simulink model "sim_quadrotor"  (R2015a)
settings: Solver=ode3  StartTime=0  StopTime=inf  FixedStep=quadEDT.sampletime  MaxStep=0.1  RelTol=1e-3
InitFcn:
  | % load parameters of the default quadrotor
  | disp('Quadrotor parameters loaded by InitFcn')
  | parameters_estimationcontrol %loads mdl_quadcopter, too!
  | 
  | % change to Simulation folder if in data folder
  | cd([matlabpath '/Simulation']);
undefined symbols (not defined in the file or in its folder): controlHelperParams, Discrete, estimParams, quad, quadEDT, Time
libraries: simulink x30, ctrlSharedLib x3, vrlib x1, commnoisgen2 x1, aerolibtransform2 x1
(part 1 of 2)
settings Model: CovSFcnEnable=off  Creator=corkep  LastModifiedBy=ra
settings DataIOCC: LimitDataPoints=off  SaveFormat=StructureWithTime  SignalLoggingSaveFormat=ModelDataLogs  SignalLogging=off  DSMLogging=off
settings OptimizationCC: ExpressionDepthLimit=2147483647  OptimizeModelRefInitCode=on  LifeSpan=1
settings DebuggingCC: UnderspecifiedInitializationDetection=Classic  MergeDetectMultiDrivingBlocksExec=none  SolverPrmCheckMsg=warning  FcnCallInpInsideContextMsg=UseLocalSettings  StateNameClashWarn=warning
settings HardwareCC: TargetBitPerLong=64  TargetBitPerPointer=64  TargetLongLongMode=on  TargetIntDivRoundTo=Zero  TargetEndianess=LittleEndian  TargetWordSize=64  TargetHWDeviceType=MATLAB Host  ProdEqTarget=off
settings RTWCC: SystemTargetFile=ert_shrlib.tlc  GenCodeOnly=on  MakeCommand="make_rtw OPTS=\"-DDEFAULT_BUFFER_SIZE=4600\""  GenerateMakefile=off  TemplateMakefile=ert_default_tmf  Description=Embedded Coder (host-based shared library target)  BuildConfiguration=Faster Runs  RTWCompilerOptimization=on
settings CodeAppCC: IgnoreCustomStorageClasses=off
settings STFCustomTargetCC: ParMdlRefBuildCompliant=on  CompOptLevelCompliant=on  IncludeMdlTerminateFcn=off  CombineOutputUpdateFcns=on  MultiInstanceERTCode=on  CodeInterfacePackaging=Reusable function  SupportVariableSizeSignals=off  ModelStepFunctionPrototypeControlCompliant=on  SystemTargetFile=ert_shrlib.tlc
settings ERTTargetCC: ParMdlRefBuildCompliant=on  CompOptLevelCompliant=on  IncludeMdlTerminateFcn=off  MultiInstanceERTCode=on  CodeInterfacePackaging=Reusable function  SupportVariableSizeSignals=off  ModelStepFunctionPrototypeControlCompliant=on  MultiInstanceErrorCode=Warning  ERTCustomFileTemplate=example_file_process.tlc

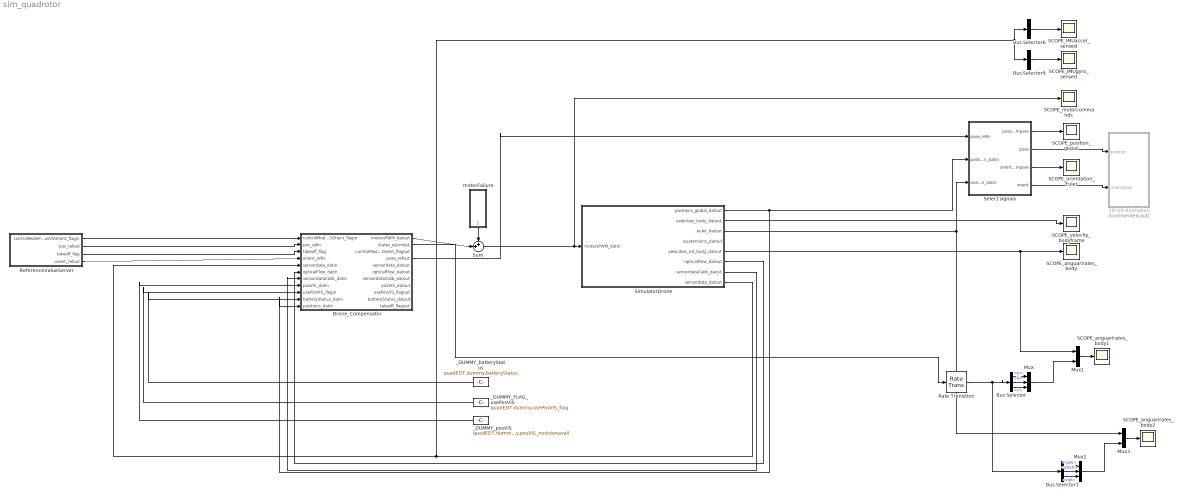
== system sim_quadrotor ==
  3D-VR-Animation : Subsystem  Commented=on
  Bus Selector : BusSelector  OutputSignals=p,q,r
  Bus Selector1 : BusSelector  OutputSignals=yaw,pitch,roll
  Bus Selector6 : BusSelector  OutputSignals=ddx,ddy,ddz  OutputAsBus=on
  Bus Selector9 : BusSelector  OutputSignals=p,q,r  OutputAsBus=on
  Drone_Compensator : Subsystem  TreatAsAtomicUnit=on
  Mux : Mux  Inputs=3
  Mux1 : Mux  Inputs=2
  Mux2 : Mux  Inputs=3
  Mux3 : Mux  Inputs=2
  Rate Transition : RateTransition
  ReferenceValueServer : Subsystem
  SCOPE_IMUaccel_sensed : Scope
      settings: TimeRange=14.995  YMin=-13  YMax=2  SaveName=ScopeData11
  SCOPE_IMUgyro_sensed : Scope
      settings: TimeRange=14.995  YMin=-0.002  YMax=0.00175  SaveName=ScopeData10
  SCOPE_anguarlrates_body : Scope
      settings: TimeRange=13.045  YMin=-1.5  YMax=0.5  SaveName=ScopeData7
  SCOPE_anguarlrates_body1 : Scope
      settings: TimeRange=13.045  YMin=-1.5  YMax=0.5  SaveName=ScopeData8
  SCOPE_anguarlrates_body2 : Scope
      settings: TimeRange=13.045  YMin=-1.5  YMax=0.5  SaveName=ScopeData13
  SCOPE_motorcommands : Scope
      settings: TimeRange=20.435  YMin=1200  YMax=1450  SaveName=ScopeData2
  SCOPE_orientation_Euler : Scope
      settings: TimeRange=29.325  YMin=-0.1  YMax=0.15  SaveName=ScopeData5
  SCOPE_position_global : Scope
      settings: TimeRange=24.935  YMin=-1.5  YMax=1  SaveName=ScopeData3
  SCOPE_velocity_bodyframe : Scope
      settings: TimeRange=13.045  YMin=-1.5  YMax=0.5  SaveName=ScopeData22
  Select signals : Subsystem
  SimulatorDrone : Subsystem
  Sum : Sum  Inputs=++|
  _DUMMY_FLAG_usePosVIS : Constant  Value=quadEDT.dummy.usePosVIS_flag
  _DUMMY_batteryStatus : Constant  Value=quadEDT.dummy.batteryStatus
  _DUMMY_posVIS : Constant  Value=quadEDT.dummy.posVIS_novisionavail
  motorFailure : Subsystem
  wires:
  Bus Selector6/1 -> SCOPE_IMUaccel_sensed/1
  Bus Selector9/1 -> SCOPE_IMUgyro_sensed/1
  ReferenceValueServer/2("pos_refout ") -> Drone_Compensator/2(pos_refin)
  motorFailure/1(motors_datout) -> Sum/1
  Drone_Compensator/1(motorsPWM_datout) -> Sum/2
  ReferenceValueServer/1(controlModePosVSOrient_flagin) -> Drone_Compensator/1(controlModePosVSOrient_flagin)
  ReferenceValueServer/4(orient_refout) -> Drone_Compensator/4(orient_refin)
  _DUMMY_posVIS/1 -> Drone_Compensator/8(posVIS_datin)
  _DUMMY_FLAG_usePosVIS/1 -> Drone_Compensator/9(usePosVIS_flagin)
  _DUMMY_batteryStatus/1 -> Drone_Compensator/10(batteryStatus_datin)
  ReferenceValueServer/3("takeoff_flag ") -> Drone_Compensator/3(takeoff_flag)
  Drone_Compensator/4(pose_refout) -> Select signals/1(pose_refin)
  Select signals/1(poseCompare) -> SCOPE_position_global/1
  Select signals/2(pose) -> 3D-VR-Animation/1(position)
  Select signals/3(orientCompare) -> SCOPE_orientation_Euler/1
  Select signals/4(orient) -> 3D-VR-Animation/2(orientation)
  SimulatorDrone/8(sensordata_datout) -> Bus Selector9/1, Bus Selector6/1, Drone_Compensator/5(sensordata_datin)
  SimulatorDrone/6(opticalFlow_datout) -> Drone_Compensator/6(opticalFlow_datin)
  SimulatorDrone/7(sensordataCalib_daout) -> Drone_Compensator/7(sensordataCalib_datin)
  SimulatorDrone/1(positions_global_datout) -> Select signals/2(position_datin), Drone_Compensator/11(positions_datin)
  SimulatorDrone/2(velocities_body_datout) -> SCOPE_velocity_bodyframe/1
  SimulatorDrone/3(euler_datout) -> Mux3/1, Select signals/3(orientation_datin)
  SimulatorDrone/5(velocities_rot_body_datout) -> Mux1/1, SCOPE_anguarlrates_body/1
  Drone_Compensator/2(states_estimout) -> Rate Transition/1
  Bus Selector/1 -> Mux/1  "<p>"
  Bus Selector/2 -> Mux/2  "<q>"
  Bus Selector/3 -> Mux/3  "<r>"
  Mux/1 -> Mux1/2
  Mux1/1 -> SCOPE_anguarlrates_body1/1
  Rate Transition/1 -> Bus Selector1/1, Bus Selector/1
  Bus Selector1/1 -> Mux2/1  "<yaw>"
  Bus Selector1/2 -> Mux2/2  "<pitch>"
  Bus Selector1/3 -> Mux2/3  "<roll>"
  Mux2/1 -> Mux3/2
  Mux3/1 -> SCOPE_anguarlrates_body2/1
  Sum/1 -> SCOPE_motorcommands/1, SimulatorDrone/1(motorsPWM_datin)

== system sim_quadrotor/3D-VR-Animation ==
  note: Student contribution by Erlend Solbakk Harbitz
  note: In animation:
      | X-axis: red
      | Y-axis: green
      | Z-axis: blue
  note: Animation
  note: Positions = [X; Y; Z] (Inertia frame with Z-axis downwards)
      | Theta      = [yaw (psi); pitch ( theta); roll (phi) ]
      |
      | Euler angles scheme: First yaw, then pitch, then roll
  position : Inport
  orientation : Inport  Port=2
  Double click for animation : vrlib/VR Sink  RequirementInfo={} %GIDa_850cb678_ba1c_4e80_94b9_fad132a707ef  InstantiateOnLoad=on  SampleTime=0.1  ViewEnable=on  RemoteChange=off  RemoteView=off  FieldsWritten=DRONE.translation.3.1.1.double#roll_rotation.rotation.4.1.1.double#pitch_rotation.rotation.4.1.1.double#yaw_rotation.rotation.4.1.1.double  WorldFileName=Animation/DroneWorld.wrl  AutoView=off  VideoDimensions=[]  AllowVariableSize=off
  Euler angle rotations : MATLAB Function  TreatAsAtomicUnit=on
  Rate Transition : RateTransition
  Rate Transition1 : RateTransition
  wires:
  orientation/1 -> Rate Transition1/1  "Euler angles (yaw, pitch, roll)"
  position/1 -> Rate Transition/1  "Inertia positions X,Y,Z"
  Rate Transition1/1 -> Euler angle rotations/1(O)
  Rate Transition/1 -> Double click for animation/1
  Euler angle rotations/1(rot_phi) -> Double click for animation/2  "Third rotation"
  Euler angle rotations/2(rot_theta) -> Double click for animation/3  "Second rotation"
  Euler angle rotations/3(rot_psi) -> Double click for animation/4  "First rotation"

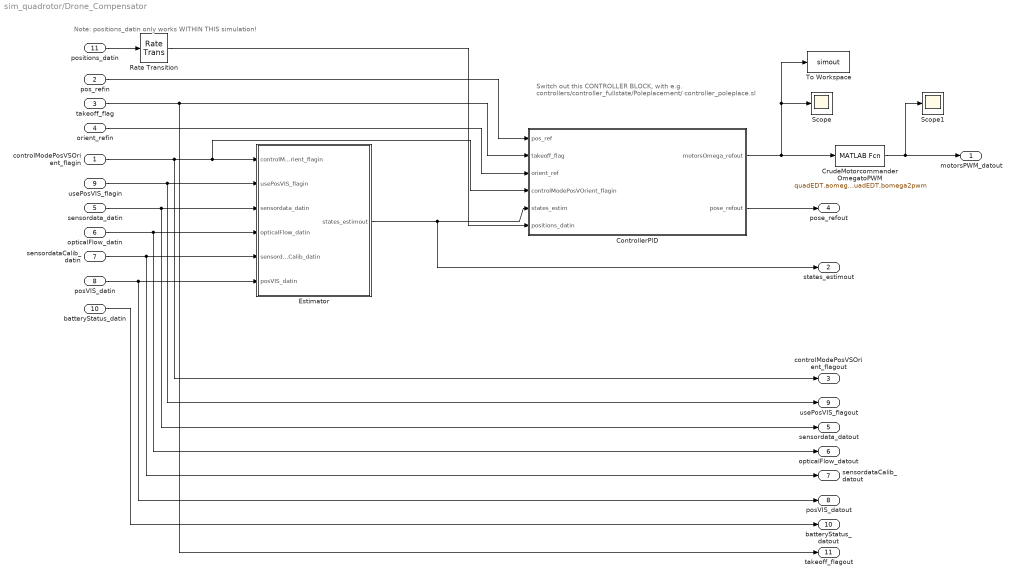
== system sim_quadrotor/Drone_Compensator ==
  note: Note: positions_datin only works WITHIN THIS simulation!
  note: Switch out this CONTROLLER BLOCK, with e.g.
      | controllers/controller_fullstate/Poleplacement/
      | controller_poleplace.sl
  controlModePosVSOrient_flagin : Inport
  pos_refin : Inport  Port=2
  takeoff_flag : Inport  Port=3
  orient_refin : Inport  Port=4
  sensordata_datin : Inport  Port=5
  opticalFlow_datin : Inport  Port=6
  sensordataCalib_datin : Inport  Port=7
  posVIS_datin : Inport  Port=8
  usePosVIS_flagin : Inport  Port=9
  batteryStatus_datin : Inport  Port=10
  positions_datin : Inport  Port=11
  ControllerPID : Subsystem  TreatAsAtomicUnit=on
  CrudeMotorcommander OmegatoPWM : MATLABFcn  MATLABFcn=quadEDT.aomega2pwm*(u-quadEDT.comega2pwm).^2+quadEDT.bomega2pwm
  Estimator : Subsystem
  Rate Transition : RateTransition
  Scope : Scope
      settings: YMin=1005  YMax=1060  SaveName=ScopeData12
  Scope1 : Scope
      settings: SaveName=ScopeData15
  To Workspace : ToWorkspace  VariableName=simout  SaveFormat=Timeseries  SampleTime=-1
  motorsPWM_datout : Outport
  states_estimout : Outport  Port=2
  controlModePosVSOrient_flagout : Outport  Port=3
  pose_refout : Outport  Port=4
  sensordata_datout : Outport  Port=5
  opticalFlow_datout : Outport  Port=6
  sensordataCalib_datout : Outport  Port=7
  posVIS_datout : Outport  Port=8
  usePosVIS_flagout : Outport  Port=9
  batteryStatus_datout : Outport  Port=10
  takeoff_flagout : Outport  Port=11
  wires:
  sensordata_datin/1 -> sensordata_datout/1, Estimator/3(sensordata_datin)
  pos_refin/1 -> ControllerPID/1(pos_ref)
  Estimator/1(states_estimout) -> ControllerPID/5(states_estim), states_estimout/1
  orient_refin/1 -> ControllerPID/3(orient_ref)
  controlModePosVSOrient_flagin/1 -> controlModePosVSOrient_flagout/1, ControllerPID/4(controlModePosVOrient_flagin), Estimator/1(controlModePosVSOrient_flagin)
  sensordataCalib_datin/1 -> sensordataCalib_datout/1, Estimator/5(sensordataCalib_datin)
  opticalFlow_datin/1 -> opticalFlow_datout/1, Estimator/4(opticalFlow_datin)
  posVIS_datin/1 -> posVIS_datout/1, Estimator/6(posVIS_datin)
  ControllerPID/1(motorsOmega_refout) -> CrudeMotorcommander OmegatoPWM/1, To Workspace/1, Scope/1
  usePosVIS_flagin/1 -> usePosVIS_flagout/1, Estimator/2(usePosVIS_flagin)
  ControllerPID/2(pose_refout) -> pose_refout/1
  batteryStatus_datin/1 -> batteryStatus_datout/1
  takeoff_flag/1 -> ControllerPID/2(takeoff_flag), takeoff_flagout/1
  positions_datin/1 -> Rate Transition/1
  Rate Transition/1 -> ControllerPID/6(positions_datin)
  CrudeMotorcommander OmegatoPWM/1 -> Scope1/1, motorsPWM_datout/1

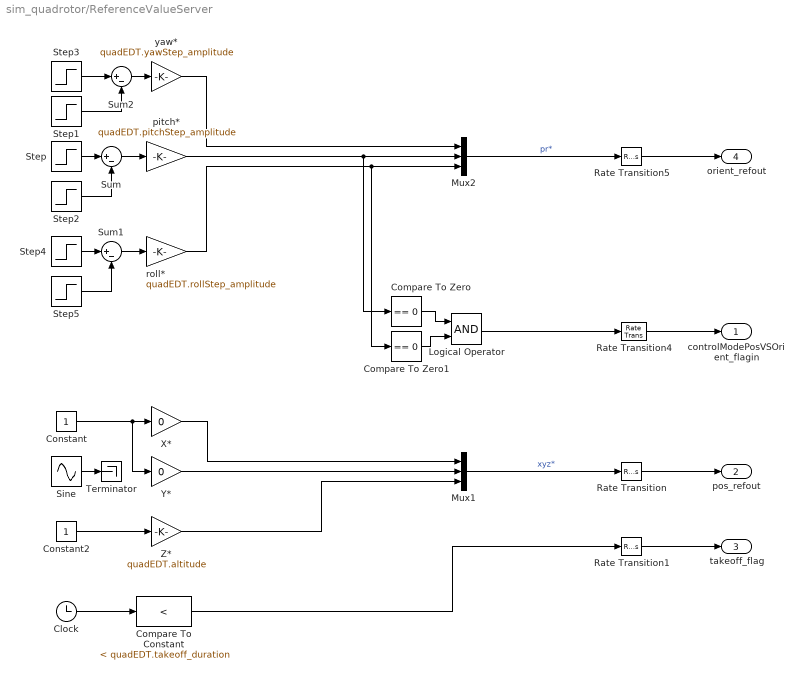
== system sim_quadrotor/ReferenceValueServer ==
  Clock : Clock
  Compare To Constant : simulink/Logic and Bit Operations/Compare To Constant  relop=<  const=quadEDT.takeoff_duration  OutDataTypeStr=boolean
  Compare To Zero : simulink/Logic and Bit Operations/Compare To Zero  relop===  OutDataTypeStr=boolean
  Compare To Zero1 : simulink/Logic and Bit Operations/Compare To Zero  relop===  OutDataTypeStr=boolean
  Constant : Constant  SampleTime=0
  Constant2 : Constant  SampleTime=0
  Logical Operator : Logic  AllPortsSameDT=off  OutDataTypeStr=boolean
  Mux1 : Mux  Inputs=3
  Mux2 : Mux  Inputs=3
  Rate Transition{,1,4..5} (4 alike) : RateTransition  OutPortSampleTime=quadEDT.sampletime
  Sine : Sin  Frequency=2*pi*.125  SampleTime=0
  Step : Step  Time=quadEDT.pitchStep_time  SampleTime=0
  Step1 : Step  Time=quadEDT.yawStep_time+quadEDT.yawStep_duration  SampleTime=0
  Step2 : Step  Time=quadEDT.pitchStep_time+quadEDT.pitchStep_duration  SampleTime=0
  Step3 : Step  Time=quadEDT.yawStep_time  SampleTime=0
  Step4 : Step  Time=quadEDT.rollStep_time  SampleTime=0
  Step5 : Step  Time=quadEDT.rollStep_duration+quadEDT.rollStep_time  SampleTime=0
  Sum : Sum  Inputs=|+-
  Sum1 : Sum  Inputs=|+-
  Sum2 : Sum  Inputs=|+-
  Terminator : Terminator
  X* : Gain  Gain=0
  Y* : Gain  Gain=0
  Z* : Gain  Gain=quadEDT.altitude
  pitch* : Gain  Gain=quadEDT.pitchStep_amplitude
  roll* : Gain  Gain=quadEDT.rollStep_amplitude
  yaw* : Gain  Gain=quadEDT.yawStep_amplitude
  controlModePosVSOrient_flagin : Outport
  "pos_refout " : Outport  Port=2
  "takeoff_flag " : Outport  Port=3
  orient_refout : Outport  Port=4
  wires:
  Y*/1 -> Mux1/2
  Constant/1 -> Y*/1, X*/1
  Mux1/1 -> Rate Transition/1  "xyz*"
  X*/1 -> Mux1/1
  Rate Transition/1 -> "pos_refout "/1
  Rate Transition4/1 -> controlModePosVSOrient_flagin/1
  Step/1 -> Sum/1
  Mux2/1 -> Rate Transition5/1  "pr*"
  Sum1/1 -> roll*/1
  Rate Transition5/1 -> orient_refout/1
  Sum/1 -> pitch*/1
  Step2/1 -> Sum/2
  yaw*/1 -> Mux2/1
  pitch*/1 -> Mux2/2, Compare To Zero/1
  roll*/1 -> Mux2/3, Compare To Zero1/1
  Compare To Zero/1 -> Logical Operator/1
  Compare To Zero1/1 -> Logical Operator/2
  Logical Operator/1 -> Rate Transition4/1
  Clock/1 -> Compare To Constant/1
  Constant2/1 -> Z*/1
  Z*/1 -> Mux1/3
  Step4/1 -> Sum1/1
  Step5/1 -> Sum1/2
  Sum2/1 -> yaw*/1
  Step3/1 -> Sum2/1
  Step1/1 -> Sum2/2
  Compare To Constant/1 -> Rate Transition1/1
  Rate Transition1/1 -> "takeoff_flag "/1
  Sine/1 -> Terminator/1

== system sim_quadrotor/Select signals ==
  pose_refin : Inport
  position_datin : Inport  Port=2
  orientation_datin : Inport  Port=3
  Mux : Mux  Inputs=2
  Mux1 : Mux  Inputs=2
  Rate Transition : RateTransition
  orientation_ref : Selector  InputPortWidth=6  Indices=[4:6]
  position_ref : Selector  InputPortWidth=6  Indices=[1:3]
  poseCompare : Outport
  pose : Outport  Port=2
  orientCompare : Outport  Port=3
  orient : Outport  Port=4
  wires:
  Rate Transition/1 -> orientation_ref/1, position_ref/1
  pose_refin/1 -> Rate Transition/1
  Mux1/1 -> orientCompare/1
  position_ref/1 -> Mux/1
  Mux/1 -> poseCompare/1
  orientation_ref/1 -> Mux1/1
  position_datin/1 -> pose/1, Mux/2
  orientation_datin/1 -> orient/1, Mux1/2

== system sim_quadrotor/SimulatorDrone ==
  motorsPWM_datin : Inport
  Bus Selector1 : BusSelector  OutputSignals=yaw,pitch,roll  OutputAsBus=on
  Bus Selector2 : BusSelector  OutputSignals=dx,dy,dz  OutputAsBus=on
  Bus Selector3 : BusSelector  OutputSignals=p,q,r  OutputAsBus=on
  Bus Selector7 : BusSelector  OutputSignals=X,Y,Z  OutputAsBus=on
  DroneRS_Sensorsystem : Subsystem
  Drone_Dynamics : Subsystem  AncestorBlock=roblocks/Dynamics/Quadrotor
  Rotation Angles to Quaternions : aerolibtransform2/Rotation Angles to Quaternions  rotationOrder=ZYX
  sensordataCalib : Constant  Value=quadEDT.sensordataCalib  SampleTime=quadEDT.sampletime
  positions_global_datout : Outport
  velocities_body_datout : Outport  Port=2
  euler_datout : Outport  Port=3
  quaternions_datout : Outport  Port=4
  velocities_rot_body_datout : Outport  Port=5
  opticalFlow_datout : Outport  Port=6
  sensordataCalib_daout : Outport  Port=7
  sensordata_datout : Outport  Port=8
  wires:
  motorsPWM_datin/1 -> Drone_Dynamics/1(motorsPwm_refin)
  Drone_Dynamics/1(states_datout) -> Bus Selector7/1, Bus Selector2/1, Bus Selector1/1, Bus Selector3/1, DroneRS_Sensorsystem/1(states_datin)
  sensordataCalib/1 -> DroneRS_Sensorsystem/2(sensordataCalib_datin)
  DroneRS_Sensorsystem/2(opticalFlow_datout) -> opticalFlow_datout/1
  DroneRS_Sensorsystem/1(sensordataCalib_datout) -> sensordataCalib_daout/1
  DroneRS_Sensorsystem/3(sensordata_datout) -> sensordata_datout/1
  Bus Selector7/1 -> positions_global_datout/1
  Bus Selector1/1 -> Rotation Angles to Quaternions/1, euler_datout/1
  Rotation Angles to Quaternions/1 -> quaternions_datout/1
  Bus Selector2/1 -> velocities_body_datout/1
  Bus Selector3/1 -> velocities_rot_body_datout/1

== system sim_quadrotor/motorFailure ==
  Mux1 : Mux
  Step : Step  Time=quadEDT.motorFailure_time  SampleTime=quadEDT.sampletime
  Step1 : Step  Time=quadEDT.motorFailure_time + quadEDT.motorFailure_duration  SampleTime=quadEDT.sampletime
  Sum : Sum  Inputs=|+-
  motorFailure_gainm1 : Gain  Gain=quadEDT.motorFailure_m2
  motorFailure_gainm2 : Gain  Gain=quadEDT.motorFailure_m2
  motorFailure_gainm3 : Gain  Gain=quadEDT.motorFailure_m3
  motorFailure_gainm4 : Gain  Gain=quadEDT.motorFailure_m3
  motors_datout : Outport
  wires:
  Step/1 -> Sum/1
  Step1/1 -> Sum/2
  Sum/1 -> motorFailure_gainm1/1, motorFailure_gainm2/1, motorFailure_gainm3/1, motorFailure_gainm4/1
  motorFailure_gainm2/1 -> Mux1/2
  motorFailure_gainm3/1 -> Mux1/3
  motorFailure_gainm4/1 -> Mux1/4
  motorFailure_gainm1/1 -> Mux1/1
  Mux1/1 -> motors_datout/1

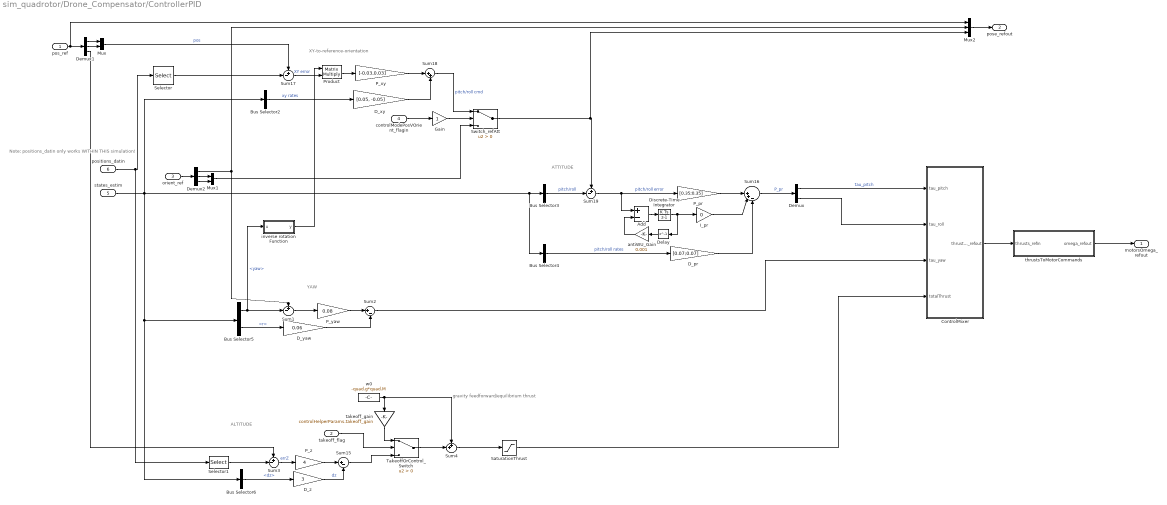
== system sim_quadrotor/Drone_Compensator/ControllerPID ==
  note: XY-to-reference-orientation
  note: ALTITUDE
  note: ATTITUDE
  note: YAW
  note: gravity feedforward/equilibrium thrust
  note: Note: positions_datin only works WITHIN THIS simulation!
  pos_ref : Inport
  takeoff_flag : Inport  Port=2
  orient_ref : Inport  Port=3
  controlModePosVOrient_flagin : Inport  Port=4
  states_estim : Inport  Port=5
  positions_datin : Inport  Port=6
  Add : Sum  Inputs=+-
  Bus Selector2 : BusSelector  OutputSignals=dx,dy  OutputAsBus=on
  Bus Selector3 : BusSelector  OutputSignals=pitch,roll  OutputAsBus=on
  Bus Selector4 : BusSelector  OutputSignals=q,p  OutputAsBus=on
  Bus Selector5 : BusSelector  OutputSignals=yaw,r
  Bus Selector6 : BusSelector  OutputSignals=dz
  ControlMixer : Subsystem
  D_pr : Gain  Gain=[0.07;0.07]
  D_xy : Gain  Gain=[0.05, -0.05]
  D_yaw : Gain  Gain=0.06
  D_z : Gain  Gain=3
  Delay : Delay  DelayLength=1  InitialCondition=0
  Demux : Demux  Outputs=2
  Demux1 : Demux  Outputs=3
  Demux2 : Demux  Outputs=3
  Discrete-Time Integrator : DiscreteIntegrator  InitialConditionSetting=State (most efficient)  SampleTime=quadEDT.sampletime  LimitOutput=on  UpperSaturationLimit=2  LowerSaturationLimit=-2
  Gain : Gain
  I_pr : Gain  Gain=0
  Mux : Mux  Inputs=2
  Mux1 : Mux  Inputs=2
  Mux2 : Mux  Inputs=3
  P_pr : Gain  Gain=[0.35;0.35]
  P_xy : Gain  Gain=[-0.03,0.03]
  P_yaw : Gain  Gain=0.08
  P_z : Gain  Gain=4
  Product : Product  Multiplication=Matrix(*)  RndMeth=Zero
  SaturationThrust : Saturate  UpperLimit=0  LowerLimit=-4*controlHelperParams.totalThrust_maxRelative*controlHelperParams.motorsThrustperMotor_max
  Selector : Selector  InputPortWidth=3  Indices=[1 2]
  Selector1 : Selector  InputPortWidth=3  Indices=[3]
  Sum{1,3,17,19} (4 alike) : Sum  Inputs=+-|
  Sum15 : Sum  Inputs=|+-
  Sum16 : Sum  Inputs=||++-
  Sum18 : Sum  Inputs=|++
  Sum2 : Sum  Inputs=|+-
  Sum4 : Sum  Inputs=++|
  Switch_refAtt : Switch  Criteria=u2 > Threshold
  TakeoffOrControl_Switch : Switch  Criteria=u2 > Threshold
  antiWU_Gain : Gain  Gain=0.001
  inverse rotation Function : MATLAB Function  TreatAsAtomicUnit=on
  takeoff_gain : Gain  Gain=controlHelperParams.takeoff_gain
  thrustsToMotorCommands : Subsystem
  w0 : Constant  Value=-quad.g*quad.M  SampleTime=quadEDT.sampletime
  motorsOmega_refout : Outport
  pose_refout : Outport  Port=2
  wires:
  w0/1 -> takeoff_gain/1, Sum4/1
  Bus Selector2/1 -> D_xy/1  "xy rates"
  Bus Selector4/1 -> D_pr/1  "pitch/roll rates"
  Sum19/1 -> P_pr/1, Add/1  "pitch/roll error"
  Sum16/1 -> Demux/1  "P_pr"
  Bus Selector5/1 -> inverse rotation Function/1(u), Sum1/2  "<yaw>"
  inverse rotation Function/1(y) -> Product/1
  Bus Selector5/2 -> D_yaw/1  "<r>"
  Sum3/1 -> P_z/1  "errZ"
  Bus Selector6/1 -> D_z/1  "<dz>"
  D_z/1 -> Sum15/2  "dz"
  D_yaw/1 -> Sum2/2
  Sum4/1 -> SaturationThrust/1
  Sum1/1 -> P_yaw/1
  Sum17/1 -> Product/2  "XY error"
  Discrete-Time Integrator/1 -> Delay/1, I_pr/1
  Demux/1 -> ControlMixer/1(tau_pitch)  "tau_pitch"
  Demux/2 -> ControlMixer/2(tau_roll)
  TakeoffOrControl_Switch/1 -> Sum4/2
  Sum15/1 -> TakeoffOrControl_Switch/3
  takeoff_gain/1 -> TakeoffOrControl_Switch/1
  Sum18/1 -> Switch_refAtt/1  "pitch/roll cmd"
  pos_ref/1 -> Mux2/1, Demux1/1
  Demux1/1 -> Mux/1
  Demux1/2 -> Mux/2
  Mux/1 -> Sum17/1  "pos"
  Demux2/2 -> Mux1/1
  Demux2/3 -> Mux1/2
  orient_ref/1 -> Demux2/1
  Mux1/1 -> Switch_refAtt/3
  Demux2/1 -> Mux2/2, Sum1/1
  Demux1/3 -> Sum3/1
  Bus Selector3/1 -> Sum19/2  "pitch/roll"
  Product/1 -> P_xy/1
  D_xy/1 -> Sum18/2
  Selector/1 -> Sum17/2
  P_z/1 -> Sum15/1
  SaturationThrust/1 -> ControlMixer/4(totalThrust)
  P_yaw/1 -> Sum2/1
  I_pr/1 -> Sum16/2
  P_pr/1 -> Sum16/1
  ControlMixer/1(thrusts_refout) -> thrustsToMotorCommands/1(thrusts_refin)
  thrustsToMotorCommands/1(omega_refout) -> motorsOmega_refout/1
  Mux2/1 -> pose_refout/1
  Switch_refAtt/1 -> Mux2/3, Sum19/1
  states_estim/1 -> Bus Selector4/1, Bus Selector3/1, Bus Selector2/1, Bus Selector5/1, Bus Selector6/1
  P_xy/1 -> Sum18/1
  Add/1 -> Discrete-Time Integrator/1
  antiWU_Gain/1 -> Add/2
  Delay/1 -> antiWU_Gain/1
  D_pr/1 -> Sum16/3
  controlModePosVOrient_flagin/1 -> Gain/1
  takeoff_flag/1 -> TakeoffOrControl_Switch/2
  Sum2/1 -> ControlMixer/3(tau_yaw)
  Gain/1 -> Switch_refAtt/2
  positions_datin/1 -> Selector1/1, Selector/1
  Selector1/1 -> Sum3/2

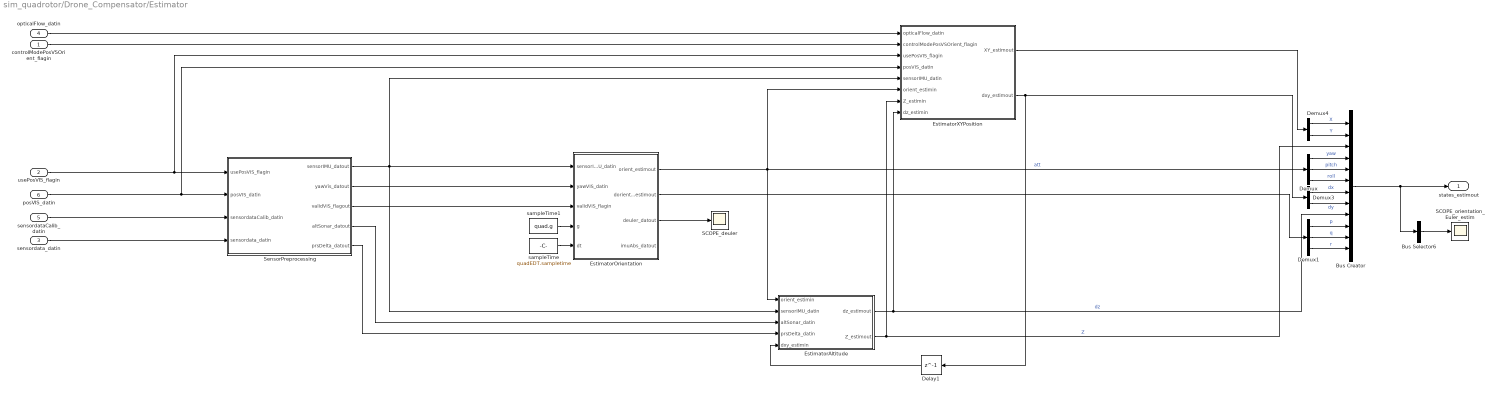
== system sim_quadrotor/Drone_Compensator/Estimator ==
  controlModePosVSOrient_flagin : Inport
  usePosVIS_flagin : Inport  Port=2
  sensordata_datin : Inport  Port=3
  opticalFlow_datin : Inport  Port=4
  sensordataCalib_datin : Inport  Port=5
  posVIS_datin : Inport  Port=6
  Bus Creator : BusCreator  Inputs='X','Y','Z','yaw','pitch','roll','dx','dy','dz','p','q','r'
  Bus Selector6 : BusSelector  OutputSignals=yaw,pitch,roll  OutputAsBus=on
  Delay1 : Delay  DelayLength=1  InitialCondition=0
  Demux : Demux  Outputs=3
  Demux1 : Demux  Outputs=3
  Demux3 : Demux  Outputs=2
  Demux4 : Demux  Outputs=2
  EstimatorAltitude : Subsystem
  EstimatorOrientation : MATLAB Function  TreatAsAtomicUnit=on
  EstimatorXYPosition : Subsystem
  SCOPE_deuler : Scope
      settings: SaveName=ScopeData6
  SCOPE_orientation_Euler_estim : Scope
      settings: TimeRange=11.74190936555891  YMin=-0.004646840148698853  YMax=0.01565055762081787  SaveName=ScopeData4
  SensorPreprocessing : Subsystem
  sampleTime : Constant  Value=quadEDT.sampletime  SampleTime=quadEDT.sampletime
  sampleTime1 : Constant  Value=quad.g  SampleTime=quadEDT.sampletime
  states_estimout : Outport
  wires:
  Bus Creator/1 -> Bus Selector6/1, states_estimout/1
  sampleTime/1 -> EstimatorOrientation/5(dt)
  sensordataCalib_datin/1 -> SensorPreprocessing/3(sensordataCalib_datin)
  EstimatorAltitude/2(Z_estimout) -> Bus Creator/3, EstimatorXYPosition/7(Z_estimin)  "Z"
  EstimatorAltitude/1(dz_estimout) -> EstimatorXYPosition/8(dz_estimin), Bus Creator/9  "dz"
  opticalFlow_datin/1 -> EstimatorXYPosition/1(opticalFlow_datin)
  Demux3/1 -> Bus Creator/7  "dx"
  Demux3/2 -> Bus Creator/8  "dy"
  EstimatorXYPosition/2(dxy_estimout) -> Delay1/1, Demux3/1
  Delay1/1 -> EstimatorAltitude/5(dxy_estimin)
  controlModePosVSOrient_flagin/1 -> EstimatorXYPosition/2(controlModePosVSOrient_flagin)
  Demux4/1 -> Bus Creator/1  "X"
  Demux4/2 -> Bus Creator/2  "Y"
  EstimatorXYPosition/1(XY_estimout) -> Demux4/1
  posVIS_datin/1 -> EstimatorXYPosition/4(posVIS_datin), SensorPreprocessing/2(posVIS_datin)
  usePosVIS_flagin/1 -> SensorPreprocessing/1(usePosVIS_flagin), EstimatorXYPosition/3(usePosVIS_flagin)
  Bus Selector6/1 -> SCOPE_orientation_Euler_estim/1
  SensorPreprocessing/1(sensorIMU_datout) -> EstimatorAltitude/2(sensorIMU_datin), EstimatorOrientation/1(sensorIMU_datin), EstimatorXYPosition/5(sensorIMU_datin)
  sensordata_datin/1 -> SensorPreprocessing/4(sensordata_datin)
  SensorPreprocessing/4(altSonar_datout) -> EstimatorAltitude/3(altSonar_datin)
  SensorPreprocessing/5(prsDelta_datout) -> EstimatorAltitude/4(prsDelta_datin)
  EstimatorOrientation/1(orient_estimout) -> EstimatorAltitude/1(orient_estimin), EstimatorXYPosition/6(orient_estimin), Demux/1  "att"
  Demux/2 -> Bus Creator/5  "pitch"
  Demux1/1 -> Bus Creator/10  "p"
  Demux1/2 -> Bus Creator/11  "q"
  Demux1/3 -> Bus Creator/12  "r"
  EstimatorOrientation/2(dorient_estimout) -> Demux1/1
  SensorPreprocessing/3(validVIS_flagout) -> EstimatorOrientation/3(validVIS_flagin)
  SensorPreprocessing/2(yawVis_datout) -> EstimatorOrientation/2(yawVIS_datin)
  Demux/3 -> Bus Creator/6  "roll"
  Demux/1 -> Bus Creator/4  "yaw"
  EstimatorOrientation/3(deuler_datout) -> SCOPE_deuler/1
  sampleTime1/1 -> EstimatorOrientation/4(g)

== system sim_quadrotor/SimulatorDrone/DroneRS_Sensorsystem ==
  states_datin : Inport
  sensordataCalib_datin : Inport  Port=2
  IMU_Pressure : Subsystem
  Rate Transition1 : RateTransition  OutPortSampleTime=quadEDT.sampletime
  camera : Subsystem
  sensordataCalib_datout : Outport
  opticalFlow_datout : Outport  Port=2
  sensordata_datout : Outport  Port=3
  wires:
  states_datin/1 -> IMU_Pressure/2(states_datin), camera/1(states_datin)
  sensordataCalib_datin/1 -> sensordataCalib_datout/1, IMU_Pressure/1(sensordataCalib_datin)
  IMU_Pressure/1(sensordata_datout) -> sensordata_datout/1
  Rate Transition1/1 -> opticalFlow_datout/1
  camera/1(opticalFlow_datout) -> Rate Transition1/1

== system sim_quadrotor/SimulatorDrone/Drone_Dynamics ==
  motorsPwm_refin : Inport
  Constant : Constant  Value=quadEDT.aomega2pwm
  Constant1 : Constant  Value=quadEDT.bomega2pwm
  Constant2 : Constant  Value=quadEDT.comega2pwm
  Directions : Gain  Gain=[1 -1 1 -1]
  Dynamics : Subsystem
  MATLAB Function : MATLAB Function  TreatAsAtomicUnit=on
  Rate Transition : RateTransition  X0=[100 100 100 100]
  omegaSaturation : Saturate  UpperLimit=quadEDT.maxomega  LowerLimit=100
  pwmSaturation : Saturate  UpperLimit=quadEDT.maxpwm  LowerLimit=quadEDT.bomega2pwm
  states_datout : Outport
  wires:
  motorsPwm_refin/1 -> pwmSaturation/1
  omegaSaturation/1 -> Directions/1
  Dynamics/1(states_datout) -> states_datout/1
  MATLAB Function/1(y) -> Rate Transition/1  "omega_ref"
  Directions/1 -> Dynamics/1(omega_refin)
  pwmSaturation/1 -> MATLAB Function/1(u)
  Constant/1 -> MATLAB Function/2(aomega2pwm)
  Constant1/1 -> MATLAB Function/3(bomega2pwm)
  Constant2/1 -> MATLAB Function/4(comega2pwm)
  Rate Transition/1 -> omegaSaturation/1

== system sim_quadrotor/Drone_Compensator/ControllerPID/ControlMixer ==
  tau_pitch : Inport
  tau_roll : Inport  Port=2
  tau_yaw : Inport  Port=3
  totalThrust : Inport  Port=4
  Mux2 : Mux
  Product : Product  Multiplication=Matrix(*)  RndMeth=Zero
  Scope : Scope
      settings: SaveName=ScopeData14
  TorquetotalThrustToThrustperMotor : Constant  Value=controlHelperParams.Q2Ts
  thrusts_refout : Outport
  wires:
  Mux2/1 -> Product/2
  TorquetotalThrustToThrustperMotor/1 -> Product/1
  totalThrust/1 -> Mux2/1
  tau_yaw/1 -> Mux2/2
  tau_pitch/1 -> Mux2/3
  tau_roll/1 -> Mux2/4
  Product/1 -> Scope/1, thrusts_refout/1

== system sim_quadrotor/Drone_Compensator/ControllerPID/thrustsToMotorCommands ==
  thrusts_refin : Inport
  Sqrt : Sqrt  SaturateOnIntegerOverflow=on
  thrustToW2 : Gain  Gain=-1/quadEDT.w2ToThrust_gain
  omega_refout : Outport
  wires:
  thrusts_refin/1 -> thrustToW2/1
  thrustToW2/1 -> Sqrt/1
  Sqrt/1 -> omega_refout/1

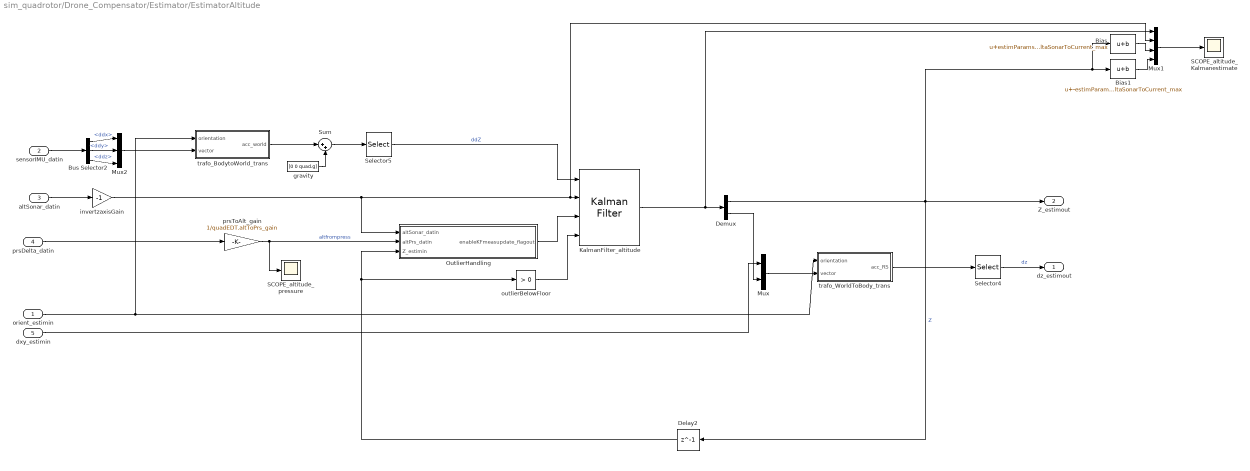
== system sim_quadrotor/Drone_Compensator/Estimator/EstimatorAltitude ==
  orient_estimin : Inport
  sensorIMU_datin : Inport  Port=2
  altSonar_datin : Inport  Port=3
  prsDelta_datin : Inport  Port=4
  dxy_estimin : Inport  Port=5
  Bias : Bias  Bias=estimParams.alt.deltaSonarToCurrent_max
  Bias1 : Bias  Bias=-estimParams.alt.deltaSonarToCurrent_max
  Bus Selector2 : BusSelector  OutputSignals=ddx,ddy,ddz
  Delay2 : Delay  DelayLength=1  InitialCondition=0
  Demux : Demux  Outputs=2
  KalmanFilter_altitude : ctrlSharedLib/Kalman Filter  TimeDomain=Discrete-Time  UseCurrentEstimator=on  ModelSource=Individual A, B, C, D matrices  ModelSourceVariable=sys  A=[1 quadEDT.sampletime; 0 1]  B=[0;quadEDT.sampletime]  C=[1 0]  D=[0]  NumberOfStates=2  NumberOfInputs=2  NumberOfOutputs=2  InitialEstimateSource=Dialog  X0=[-0.046 0]  P0=10  UseK=off  UseGH=on  NumberOfProcessNoiseInputs=2  G=estimParams.alt.kf.G  TimeInvariantG=on  H=estimParams.alt.kf.H  TimeInvariantH=on  Q=estimParams.alt.kf.Q  TimeInvariantQ=on  R=estimParams.alt.kf.R  TimeInvariantR=on  N=estimParams.alt.kf.N  TimeInvariantN=on  AddInputPort=on  AddEnablePort=on  ExternalReset=Level hold  OutputEstimatedY=off  OutputP=off  Ts=-1
  Mux : Mux  Inputs=2
  Mux1 : Mux
  Mux2 : Mux  Inputs=3
  OutlierHandling : Subsystem
  SCOPE_altitude_Kalmanestimate : Scope
      settings: TimeRange=13  YMax=1  SaveName=ScopeData25
  SCOPE_altitude_pressure : Scope
      settings: TimeRange=10  YMin=-1  YMax=0.4000000000000001  SaveName=ScopeData9
  Selector4 : Selector  InputPortWidth=3  Indices=[3]
  Selector5 : Selector  InputPortWidth=3  Indices=[3]
  Sum : Sum  Inputs=|++
  gravity : Constant  Value=[0 0 quad.g]
  invertzaxisGain : Gain  Gain=-1
  outlierBelowFloor : simulink/Logic and Bit Operations/Compare To Constant  relop=>  const=0  OutDataTypeStr=boolean
  prsToAlt_gain : Gain  Gain=1/quadEDT.altToPrs_gain
  trafo_BodytoWorld_trans : MATLAB Function  TreatAsAtomicUnit=on
  trafo_WorldToBody_trans : MATLAB Function  TreatAsAtomicUnit=on
  dz_estimout : Outport
  Z_estimout : Outport  Port=2
  wires:
  orient_estimin/1 -> trafo_BodytoWorld_trans/1(orientation), trafo_WorldToBody_trans/1(orientation)
  altSonar_datin/1 -> invertzaxisGain/1
  trafo_BodytoWorld_trans/1(acc_world) -> Sum/1
  gravity/1 -> Sum/2
  Sum/1 -> Selector5/1
  KalmanFilter_altitude/1 -> Mux1/1, Demux/1
  Mux/1 -> trafo_WorldToBody_trans/2(vector)
  Selector5/1 -> KalmanFilter_altitude/1  "ddZ"
  invertzaxisGain/1 -> Mux1/2, KalmanFilter_altitude/2, OutlierHandling/1(altSonar_datin)
  Demux/1 -> Bias1/1, Bias/1, Delay2/1, Z_estimout/1  "Z"
  Selector4/1 -> dz_estimout/1  "dz"
  Demux/2 -> Mux/2
  Mux1/1 -> SCOPE_altitude_Kalmanestimate/1
  Bias/1 -> Mux1/3
  Bias1/1 -> Mux1/4
  outlierBelowFloor/1 -> KalmanFilter_altitude/4
  prsDelta_datin/1 -> prsToAlt_gain/1
  prsToAlt_gain/1 -> SCOPE_altitude_pressure/1, OutlierHandling/2(altPrs_datin)  "altfrompress"
  Delay2/1 -> outlierBelowFloor/1, OutlierHandling/3(Z_estimin)
  OutlierHandling/1(enableKFmeasupdate_flagout) -> KalmanFilter_altitude/3
  dxy_estimin/1 -> Mux/1
  trafo_WorldToBody_trans/1(acc_RS) -> Selector4/1
  Bus Selector2/1 -> Mux2/1  "<ddx>"
  Bus Selector2/2 -> Mux2/2  "<ddy>"
  Bus Selector2/3 -> Mux2/3  "<ddz>"
  sensorIMU_datin/1 -> Bus Selector2/1
  Mux2/1 -> trafo_BodytoWorld_trans/2(vector)

== system sim_quadrotor/Drone_Compensator/Estimator/EstimatorXYPosition ==
  opticalFlow_datin : Inport
  controlModePosVSOrient_flagin : Inport  Port=2
  usePosVIS_flagin : Inport  Port=3
  posVIS_datin : Inport  Port=4
  sensorIMU_datin : Inport  Port=5
  orient_estimin : Inport  Port=6
  Z_estimin : Inport  Port=7
  dz_estimin : Inport  Port=8
  EstimatorVelocity : Subsystem
  EstimatorXYPosition : Subsystem
  XY_estimout : Outport
  dxy_estimout : Outport  Port=2
  wires:
  orient_estimin/1 -> EstimatorVelocity/4(orient_estimin), EstimatorXYPosition/2(orient_estimin)
  EstimatorVelocity/1(dxy_estimout) -> EstimatorXYPosition/1(dxy_estimin), dxy_estimout/1
  opticalFlow_datin/1 -> EstimatorVelocity/1(opticalFlow_datin)
  sensorIMU_datin/1 -> EstimatorVelocity/3(sensorIMU_datin)
  Z_estimin/1 -> EstimatorVelocity/2(Z_estimin)
  controlModePosVSOrient_flagin/1 -> EstimatorXYPosition/3(controlModePosVSOrient_flagin)
  dz_estimin/1 -> EstimatorXYPosition/4(dz_estimin)
  posVIS_datin/1 -> EstimatorXYPosition/5(posVIS_datin)
  usePosVIS_flagin/1 -> EstimatorXYPosition/6(usePosVIS_flagin)
  EstimatorXYPosition/1(XY_estimout) -> XY_estimout/1

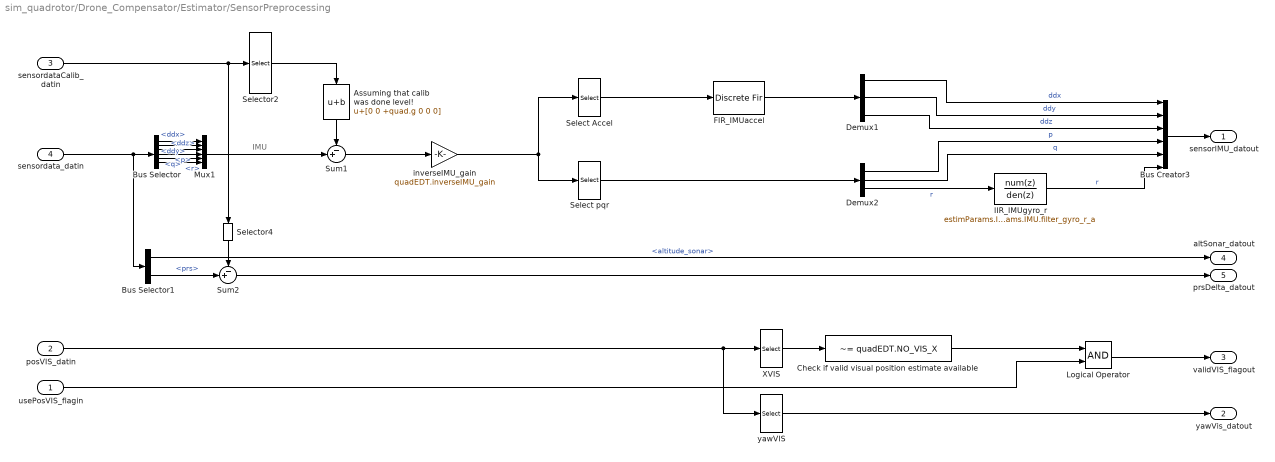
== system sim_quadrotor/Drone_Compensator/Estimator/SensorPreprocessing ==
  note: IMU
  usePosVIS_flagin : Inport
  posVIS_datin : Inport  Port=2
  sensordataCalib_datin : Inport  Port=3
  sensordata_datin : Inport  Port=4
  Assuming that calib was done level! : Bias  Bias=[0 0 +quad.g 0 0 0]
  Bus Creator3 : BusCreator  Inputs=6
  Bus Selector : BusSelector  OutputSignals=ddx,ddy,ddz,p,q,r
  Bus Selector1 : BusSelector  OutputSignals=altitude_sonar,prs
  Check if valid visual position estimate available : simulink/Logic and Bit Operations/Compare To Constant  relop=~=  const=quadEDT.NO_VIS_X  OutDataTypeStr=boolean
  Demux1 : Demux  Outputs=3
  Demux2 : Demux  Outputs=3
  FIR_IMUaccel : DiscreteFir  Coefficients=estimParams.IMU.filter_accel.Coefficients
  IIR_IMUgyro_r : DiscreteFilter  Numerator=estimParams.IMU.filter_gyro_r_b  Denominator=estimParams.IMU.filter_gyro_r_a
  Logical Operator : Logic  AllPortsSameDT=off  OutDataTypeStr=boolean
  Mux1 : Mux  Inputs=6
  Select Accel : Selector  InputPortWidth=6  Indices=[1 2 3]
  Select pqr : Selector  InputPortWidth=6  Indices=[4 5 6]
  Selector2 : Selector  InputPortWidth=7  Indices=[1:6]
  Selector4 : Selector  InputPortWidth=7  Indices=[7]
  Sum1 : Sum  Inputs=-+|
  Sum2 : Sum  Inputs=-+|
  XVIS : Selector  InputPortWidth=4
  inverseIMU_gain : Gain  Gain=quadEDT.inverseIMU_gain
  yawVIS : Selector  InputPortWidth=4  Indices=4
  sensorIMU_datout : Outport
  yawVis_datout : Outport  Port=2
  validVIS_flagout : Outport  Port=3
  altSonar_datout : Outport  Port=4
  prsDelta_datout : Outport  Port=5
  wires:
  posVIS_datin/1 -> yawVIS/1, XVIS/1
  Bus Creator3/1 -> sensorIMU_datout/1
  Demux1/1 -> Bus Creator3/1  "ddx"
  Demux1/2 -> Bus Creator3/2  "ddy"
  Demux1/3 -> Bus Creator3/3  "ddz"
  Sum1/1 -> inverseIMU_gain/1
  Selector2/1 -> Assuming that calib was done level!/1
  Demux2/1 -> Bus Creator3/4  "p"
  Demux2/2 -> Bus Creator3/5  "q"
  inverseIMU_gain/1 -> Select pqr/1, Select Accel/1
  Select Accel/1 -> FIR_IMUaccel/1
  FIR_IMUaccel/1 -> Demux1/1
  Demux2/3 -> IIR_IMUgyro_r/1  "r"
  IIR_IMUgyro_r/1 -> Bus Creator3/6  "r"
  sensordataCalib_datin/1 -> Selector4/1, Selector2/1
  Bus Selector/1 -> Mux1/1  "<ddx>"
  Bus Selector/2 -> Mux1/2  "<ddy>"
  Bus Selector/3 -> Mux1/3  "<ddz>"
  Bus Selector/4 -> Mux1/4  "<p>"
  Bus Selector/5 -> Mux1/5  "<q>"
  Bus Selector/6 -> Mux1/6  "<r>"
  sensordata_datin/1 -> Bus Selector1/1, Bus Selector/1
  Bus Selector1/1 -> altSonar_datout/1  "<altitude_sonar>"
  Selector4/1 -> Sum2/1
  Bus Selector1/2 -> Sum2/2  "<prs>"
  Sum2/1 -> prsDelta_datout/1
  Mux1/1 -> Sum1/2
  XVIS/1 -> Check if valid visual position estimate available/1
  yawVIS/1 -> yawVis_datout/1
  Logical Operator/1 -> validVIS_flagout/1
  Check if valid visual position estimate available/1 -> Logical Operator/1
  usePosVIS_flagin/1 -> Logical Operator/2
  Assuming that calib was done level!/1 -> Sum1/1
  Select pqr/1 -> Demux2/1

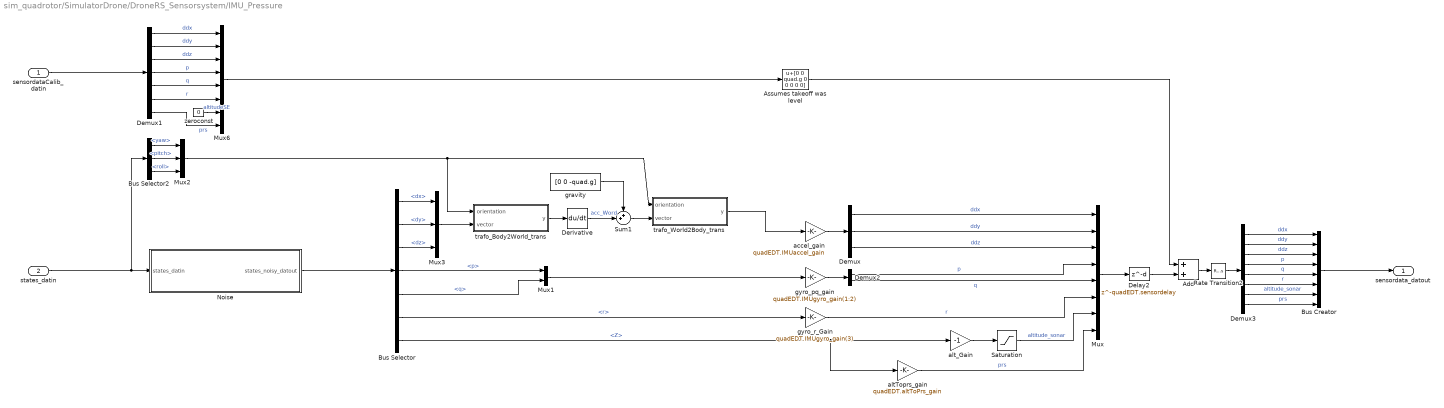
== system sim_quadrotor/SimulatorDrone/DroneRS_Sensorsystem/IMU_Pressure ==
  sensordataCalib_datin : Inport
  states_datin : Inport  Port=2
  " Noise" : Subsystem
  Add : Sum
  Assumes takeoff was level : Bias  Bias=[0 0 quad.g 0 0 0 0 0]
  Bus Creator : BusCreator  Inputs=8
  Bus Selector : BusSelector  OutputSignals=dx,dy,dz,p,q,r,Z
  Bus Selector2 : BusSelector  OutputSignals=yaw,pitch,roll
  Delay2 : Delay  DelayLength=quadEDT.sensordelay  InitialCondition=[quadEDT.sensordataCalib(1:6),0,quadEDT.sensordataCalib(7)]
  Demux : Demux  Outputs=3
  Demux1 : Demux  Outputs=7
  Demux2 : Demux  Outputs=2
  Demux3 : Demux  Outputs=8
  Derivative : Derivative
  Mux : Mux  Inputs=8
  Mux1 : Mux  Inputs=2
  Mux2 : Mux  Inputs=3
  Mux3 : Mux  Inputs=3
  Mux6 : Mux  Inputs=8
  Rate Transition2 : RateTransition  X0=[quadEDT.sensordataCalib(1:6),0,quadEDT.sensordataCalib(7)]  OutPortSampleTime=quadEDT.sampletime
  Saturation : Saturate  UpperLimit=inf  LowerLimit=quadEDT.altSenor_min
  Sum1 : Sum  Inputs=++|
  accel_gain : Gain  Gain=quadEDT.IMUaccel_gain
  altToprs_gain : Gain  Gain=quadEDT.altToPrs_gain
  alt_Gain : Gain  Gain=-1
  gravity : Constant  Value=[0 0 -quad.g]
  gyro_pq_gain : Gain  Gain=quadEDT.IMUgyro_gain(1:2)
  gyro_r_Gain : Gain  Gain=quadEDT.IMUgyro_gain(3)
  trafo_Body2World_trans : MATLAB Function  TreatAsAtomicUnit=on
  trafo_World2Body_trans : MATLAB Function  TreatAsAtomicUnit=on
  zeroconst : Constant  Value=0
  sensordata_datout : Outport
  wires:
  states_datin/1 -> " Noise"/1(states_datin), Bus Selector2/1
  sensordataCalib_datin/1 -> Demux1/1
  Demux2/2 -> Mux/5  "q"
  Demux2/1 -> Mux/4  "p"
  " Noise"/1(states_noisy_datout) -> Bus Selector/1
  Bus Selector/2 -> Mux3/2  "<dy>"
  trafo_World2Body_trans/1(y) -> accel_gain/1
  Demux/1 -> Mux/1  "ddx"
  Demux/2 -> Mux/2  "ddy"
  gyro_r_Gain/1 -> Mux/6  "r"
  Bus Selector2/1 -> Mux2/1  "<yaw>"
  Bus Selector2/2 -> Mux2/2  "<pitch>"
  Bus Selector2/3 -> Mux2/3  "<roll>"
  Demux/3 -> Mux/3  "ddz"
  Mux2/1 -> trafo_Body2World_trans/1(orientation), trafo_World2Body_trans/1(orientation)
  gravity/1 -> Sum1/1
  Bus Selector/4 -> Mux1/1  "<p>"
  Bus Selector/5 -> Mux1/2  "<q>"
  Bus Selector/6 -> gyro_r_Gain/1  "<r>"
  Bus Selector/7 -> altToprs_gain/1, alt_Gain/1  "<Z>"
  alt_Gain/1 -> Saturation/1
  Saturation/1 -> Mux/7  "altitude_sonar"
  Bus Selector/3 -> Mux3/3  "<dz>"
  altToprs_gain/1 -> Mux/8  "prs"
  Demux1/1 -> Mux6/1  "ddx"
  Demux1/2 -> Mux6/2  "ddy"
  Demux1/3 -> Mux6/3  "ddz"
  Demux1/4 -> Mux6/4  "p"
  Demux1/5 -> Mux6/5  "q"
  Demux1/6 -> Mux6/6  "r"
  zeroconst/1 -> Mux6/7  "altitudeSE"
  Demux1/7 -> Mux6/8  "prs"
  Mux6/1 -> Assumes takeoff was level/1
  Add/1 -> Rate Transition2/1
  Mux/1 -> Delay2/1
  Demux3/3 -> Bus Creator/3  "ddz"
  Demux3/1 -> Bus Creator/1  "ddx"
  Demux3/2 -> Bus Creator/2  "ddy"
  Demux3/4 -> Bus Creator/4  "p"
  Demux3/5 -> Bus Creator/5  "q"
  Demux3/6 -> Bus Creator/6  "r"
  Demux3/7 -> Bus Creator/7  "altitude_sonar"
  Demux3/8 -> Bus Creator/8  "prs"
  Bus Creator/1 -> sensordata_datout/1
  Mux1/1 -> gyro_pq_gain/1
  Bus Selector/1 -> Mux3/1  "<dx>"
  Delay2/1 -> Add/2
  accel_gain/1 -> Demux/1
  gyro_pq_gain/1 -> Demux2/1
  Mux3/1 -> trafo_Body2World_trans/2(vector)
  trafo_Body2World_trans/1(y) -> Derivative/1
  Sum1/1 -> trafo_World2Body_trans/2(vector)
  Derivative/1 -> Sum1/2  "acc_Word"
  Assumes takeoff was level/1 -> Add/1
  Rate Transition2/1 -> Demux3/1

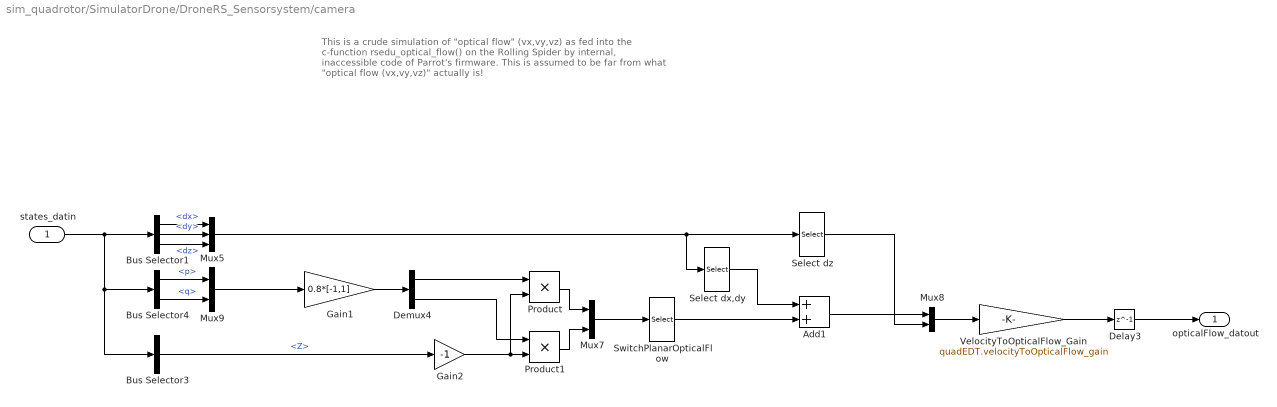
== system sim_quadrotor/SimulatorDrone/DroneRS_Sensorsystem/camera ==
  note: This is a crude simulation of "optical flow" (vx,vy,vz) as
      | fed into the c-function rsedu_optical_flow() on the Rolling Spider
      | by internal, inaccessible code of Parrot's firmware.
      | This is assumed to be far from what "optical flow (vx,vy,vz)" actually is!
  states_datin : Inport
  Add1 : Sum
  Bus Selector1 : BusSelector  OutputSignals=dx,dy,dz
  Bus Selector3 : BusSelector  OutputSignals=Z
  Bus Selector4 : BusSelector  OutputSignals=p,q
  Delay3 : Delay  DelayLength=1  InitialCondition=0
  Demux4 : Demux  Outputs=2
  Gain1 : Gain  Gain=0.8*[-1,1]
  Gain2 : Gain  Gain=-1
  Mux5 : Mux  Inputs=3
  Mux7 : Mux  Inputs=2
  Mux8 : Mux  Inputs=2
  Mux9 : Mux  Inputs=2
  Product : Product
  Product1 : Product
  Select dx,dy : Selector  InputPortWidth=3  Indices=[1 2]
  Select dz : Selector  InputPortWidth=3  Indices=3
  SwitchPlanarOpticalFlow : Selector  InputPortWidth=2  Indices=[2 1]
  VelocityToOpticalFlow_Gain : Gain  Gain=quadEDT.velocityToOpticalFlow_gain
  opticalFlow_datout : Outport
  wires:
  states_datin/1 -> Bus Selector3/1, Bus Selector4/1, Bus Selector1/1
  Bus Selector1/1 -> Mux5/1  "<dx>"
  Bus Selector1/2 -> Mux5/2  "<dy>"
  Bus Selector1/3 -> Mux5/3  "<dz>"
  VelocityToOpticalFlow_Gain/1 -> Delay3/1
  Mux5/1 -> Select dx,dy/1, Select dz/1
  Demux4/1 -> Product/1
  Gain1/1 -> Demux4/1
  Demux4/2 -> Product1/1
  Product/1 -> Mux7/1
  Product1/1 -> Mux7/2
  Mux7/1 -> SwitchPlanarOpticalFlow/1
  Mux9/1 -> Gain1/1
  Gain2/1 -> Product/2, Product1/2
  Select dx,dy/1 -> Add1/1
  SwitchPlanarOpticalFlow/1 -> Add1/2
  Add1/1 -> Mux8/1
  Select dz/1 -> Mux8/2
  Bus Selector3/1 -> Gain2/1  "<Z>"
  Bus Selector4/1 -> Mux9/1  "<p>"
  Bus Selector4/2 -> Mux9/2  "<q>"
  Mux8/1 -> VelocityToOpticalFlow_Gain/1
  Delay3/1 -> opticalFlow_datout/1

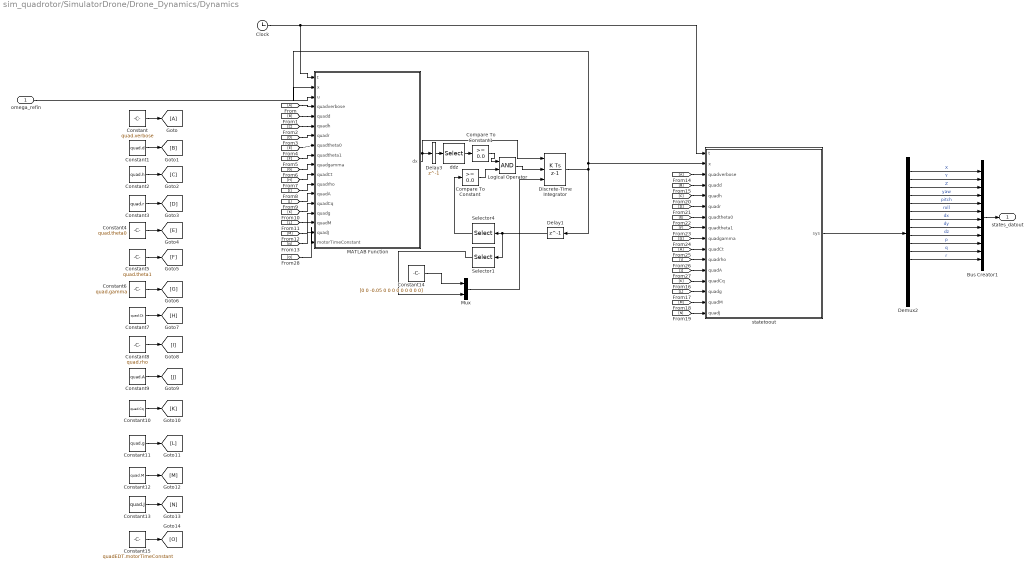
== system sim_quadrotor/SimulatorDrone/Drone_Dynamics/Dynamics ==
  omega_refin : Inport
  Bus Creator1 : BusCreator  Inputs='X','Y','Z','yaw','pitch','roll','dx','dy','dz','p','q','r'
  Clock : Clock
  Compare To Constant : simulink/Logic and Bit Operations/Compare To Constant  relop=>=  const=0.0  OutDataTypeStr=uint8
  Compare To Constant1 : simulink/Logic and Bit Operations/Compare To Constant  relop=>=  const=0.0  OutDataTypeStr=uint8
  Constant : Constant  Value=quad.verbose
  Constant1 : Constant  Value=quad.d
  Constant10 : Constant  Value=quad.Cq
  Constant11 : Constant  Value=quad.g
  Constant12 : Constant  Value=quad.M
  Constant13 : Constant  Value=quad.J
  Constant14 : Constant  Value=[0 0 -0.05 0 0 0 0 0 0 0 0 0]
  Constant15 : Constant  Value=quadEDT.motorTimeConstant
  Constant2 : Constant  Value=quad.h
  Constant3 : Constant  Value=quad.r
  Constant4 : Constant  Value=quad.theta0
  Constant5 : Constant  Value=quad.theta1
  Constant6 : Constant  Value=quad.gamma
  Constant7 : Constant  Value=quad.Ct
  Constant8 : Constant  Value=quad.rho
  Constant9 : Constant  Value=quad.A
  Delay1 : Delay  DelayLength=1  InitialCondition=[0 0 0 0 0 0 0 0 0 0 0 0 200 -200 200 -200]
  Delay3 : Delay  DelayLength=1  InitialCondition=0
  Demux2 : Demux  Outputs=16
  Discrete-Time Integrator : DiscreteIntegrator  ExternalReset=level  InitialConditionSource=external  InitialConditionSetting=State (most efficient)  SampleTime=quadEDT.sampletime
  Logical Operator : Logic  AllPortsSameDT=off  OutDataTypeStr=boolean
  MATLAB Function : MATLAB Function  TreatAsAtomicUnit=on
  Mux : Mux  Inputs=2
  Selector1 : Selector  InputPortWidth=16  Indices=[13:16]
  Selector4 : Selector  InputPortWidth=16  Indices=3
  ddz : Selector  InputPortWidth=16  Indices=9
  statetoout : MATLAB Function  TreatAsAtomicUnit=on
  states_datout : Outport
  wires:
  Demux2/3 -> Bus Creator1/3  "Z"
  Demux2/1 -> Bus Creator1/1  "X"
  Demux2/5 -> Bus Creator1/5  "pitch"
  Demux2/4 -> Bus Creator1/4  "yaw"
  Demux2/7 -> Bus Creator1/7  "dx"
  Demux2/9 -> Bus Creator1/9  "dz"
  Demux2/2 -> Bus Creator1/2  "Y"
  Demux2/6 -> Bus Creator1/6  "roll"
  Demux2/8 -> Bus Creator1/8  "dy"
  Discrete-Time Integrator/1 -> Delay1/1, MATLAB Function/2(x), statetoout/2(x)
  Bus Creator1/1 -> states_datout/1
  Demux2/10 -> Bus Creator1/10  "p"
  Demux2/11 -> Bus Creator1/11  "q"
  Demux2/12 -> Bus Creator1/12  "r"
  omega_refin/1 -> MATLAB Function/3(u)
  MATLAB Function/1(dx) -> Delay3/1, Discrete-Time Integrator/1
  Clock/1 -> MATLAB Function/1(t), statetoout/1(t)
  Constant9/1 -> [J]
  Constant/1 -> [A]
  Constant10/1 -> [K]
  Constant1/1 -> [B]
  Constant13/1 -> [N]
  Constant2/1 -> [C]
  Constant5/1 -> [F]
  Constant3/1 -> [D]
  [N] -> statetoout/16(quadJ)
  Constant4/1 -> [E]
  Constant7/1 -> [H]
  Constant6/1 -> [G]
  Constant8/1 -> [I]
  Constant12/1 -> [M]
  Constant11/1 -> [L]
  [B] -> MATLAB Function/5(quadd)
  [A] -> MATLAB Function/4(quadverbose)
  [C] -> MATLAB Function/6(quadh)
  [E] -> MATLAB Function/8(quadtheta0)
  [D] -> MATLAB Function/7(quadr)
  [F] -> MATLAB Function/9(quadtheta1)
  [H] -> MATLAB Function/11(quadCt)
  [G] -> MATLAB Function/10(quadgamma)
  [I] -> MATLAB Function/12(quadrho)
  [K] -> MATLAB Function/14(quadCq)
  [J] -> MATLAB Function/13(quadA)
  [L] -> MATLAB Function/15(quadg)
  [M] -> MATLAB Function/16(quadM)
  [N] -> MATLAB Function/17(quadJ)
  [A] -> statetoout/3(quadverbose)
  statetoout/1(sys) -> Demux2/1
  [B] -> statetoout/4(quadd)
  [D] -> statetoout/6(quadr)
  [C] -> statetoout/5(quadh)
  [E] -> statetoout/7(quadtheta0)
  [G] -> statetoout/9(quadgamma)
  [F] -> statetoout/8(quadtheta1)
  [H] -> statetoout/10(quadCt)
  [J] -> statetoout/12(quadA)
  [I] -> statetoout/11(quadrho)
  [K] -> statetoout/13(quadCq)
  [L] -> statetoout/14(quadg)
  [M] -> statetoout/15(quadM)
  Selector4/1 -> Compare To Constant/1
  Compare To Constant/1 -> Logical Operator/2
  Logical Operator/1 -> Discrete-Time Integrator/2
  ddz/1 -> Compare To Constant1/1
  Compare To Constant1/1 -> Logical Operator/1
  Delay3/1 -> ddz/1
  Mux/1 -> Discrete-Time Integrator/3
  Constant15/1 -> [O]
  [O] -> MATLAB Function/18(motorTimeConstant)
  Constant14/1 -> Mux/1
  Delay1/1 -> Selector1/1, Selector4/1
  Selector1/1 -> Mux/2

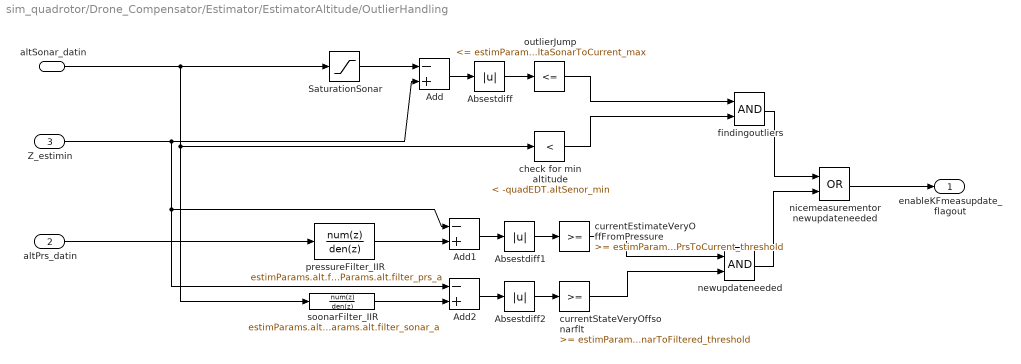
== system sim_quadrotor/Drone_Compensator/Estimator/EstimatorAltitude/OutlierHandling ==
  altSonar_datin : Inport
  altPrs_datin : Inport  Port=2
  Z_estimin : Inport  Port=3
  Absestdiff : Abs
  Absestdiff1 : Abs
  Absestdiff2 : Abs
  Add : Sum  Inputs=-+
  Add1 : Sum  Inputs=-+
  Add2 : Sum  Inputs=-+
  SaturationSonar : Saturate  UpperLimit=-quadEDT.altSenor_min  LowerLimit=-inf
  check for min altitude : simulink/Logic and Bit Operations/Compare To Constant  relop=<  const=-quadEDT.altSenor_min  OutDataTypeStr=boolean
  currentEstimateVeryOffFromPressure : simulink/Logic and Bit Operations/Compare To Constant  relop=>=  const=estimParams.alt.deltaPrsToCurrent_threshold  OutDataTypeStr=boolean
  currentStateVeryOffsonarflt : simulink/Logic and Bit Operations/Compare To Constant  relop=>=  const=estimParams.alt.deltaSonarToFiltered_threshold  OutDataTypeStr=boolean
  findingoutliers : Logic  AllPortsSameDT=off  OutDataTypeStr=boolean
  newupdateneeded : Logic  AllPortsSameDT=off  OutDataTypeStr=boolean
  nicemeasurementor newupdateneeded : Logic  Operator=OR  AllPortsSameDT=off  OutDataTypeStr=boolean
  outlierJump : simulink/Logic and Bit Operations/Compare To Constant  relop=<=  const=estimParams.alt.deltaSonarToCurrent_max  OutDataTypeStr=boolean
  pressureFilter_IIR : DiscreteFilter  Numerator=estimParams.alt.filter_prs_b  Denominator=estimParams.alt.filter_prs_a
  soonarFilter_IIR : DiscreteFilter  Numerator=estimParams.alt.filter_sonar_b  Denominator=estimParams.alt.filter_sonar_a
  enableKFmeasupdate_flagout : Outport
  wires:
  Absestdiff1/1 -> currentEstimateVeryOffFromPressure/1
  soonarFilter_IIR/1 -> Add2/2
  altPrs_datin/1 -> pressureFilter_IIR/1
  pressureFilter_IIR/1 -> Add1/2
  currentStateVeryOffsonarflt/1 -> newupdateneeded/2
  Add2/1 -> Absestdiff2/1
  Z_estimin/1 -> Add/2, Add2/1, Add1/1
  currentEstimateVeryOffFromPressure/1 -> newupdateneeded/1
  altSonar_datin/1 -> check for min altitude/1, soonarFilter_IIR/1, SaturationSonar/1
  Absestdiff2/1 -> currentStateVeryOffsonarflt/1
  newupdateneeded/1 -> nicemeasurementor newupdateneeded/2
  Add/1 -> Absestdiff/1
  Absestdiff/1 -> outlierJump/1
  SaturationSonar/1 -> Add/1
  outlierJump/1 -> findingoutliers/1
  check for min altitude/1 -> findingoutliers/2
  findingoutliers/1 -> nicemeasurementor newupdateneeded/1
  nicemeasurementor newupdateneeded/1 -> enableKFmeasupdate_flagout/1
  Add1/1 -> Absestdiff1/1

== system sim_quadrotor/Drone_Compensator/Estimator/EstimatorXYPosition/EstimatorVelocity ==
  opticalFlow_datin : Inport
  Z_estimin : Inport  Port=2
  sensorIMU_datin : Inport  Port=3
  orient_estimin : Inport  Port=4
  AccelerationHandling : Subsystem
  Delay : Delay  DelayLength=1  InitialCondition=0
  KalmanFilter_dxdy : ctrlSharedLib/Kalman Filter  TimeDomain=Discrete-Time  UseCurrentEstimator=on  ModelSource=Individual A, B, C, D matrices  ModelSourceVariable=ss(0.95,1,1,0,1)  A=eye(2)  B=quadEDT.sampletime*eye(2)  C=eye(2)  D=0  NumberOfStates=1  NumberOfInputs=1  NumberOfOutputs=1  InitialEstimateSource=Dialog  X0=0  P0=10  UseK=off  UseGH=on  NumberOfProcessNoiseInputs=1  G=estimParams.pos.kfvelo.G  TimeInvariantG=on  H=estimParams.pos.kfvelo.H  TimeInvariantH=on  Q=estimParams.pos.kfvelo.Q  TimeInvariantQ=on  R=estimParams.pos.kfvelo.R  TimeInvariantR=on  N=estimParams.pos.kfvelo.N  TimeInvariantN=on  AddInputPort=on  AddEnablePort=on  OutputEstimatedY=off  OutputP=off  Ts=-1
  Mux : Mux  Inputs=2
  SCOPE_dxy : Scope
      settings: TimeRange=2.5  YMin=-12  YMax=6
  SCOPE_enableKFdxyupdate : Scope
      settings: TimeRange=2.2  YMin=0  YMax=1
  Select dxy : Selector  InputPortWidth=3  Indices=[1 2]
  UglyDataHandling : Subsystem
  opticalFlowToVelocity_gain : Gain  Gain=estimParams.pos.opticalFlowToVelocity_gain
  dxy_estimout : Outport
  wires:
  orient_estimin/1 -> AccelerationHandling/2(orient_estimin), UglyDataHandling/1(orient_estimin)
  sensorIMU_datin/1 -> AccelerationHandling/3(sensorIMU_datin), UglyDataHandling/2(sensorIMU_datin)
  opticalFlow_datin/1 -> opticalFlowToVelocity_gain/1
  Select dxy/1 -> AccelerationHandling/1(dxy_estimin), UglyDataHandling/4(dxy_estimin), KalmanFilter_dxdy/2, Mux/1
  opticalFlowToVelocity_gain/1 -> Select dxy/1
  KalmanFilter_dxdy/1 -> Mux/2, dxy_estimout/1, Delay/1
  UglyDataHandling/1(enable_flag) -> SCOPE_enableKFdxyupdate/1, KalmanFilter_dxdy/3
  Z_estimin/1 -> AccelerationHandling/4(Z_estimin), UglyDataHandling/3(Z_estimin)
  Mux/1 -> SCOPE_dxy/1
  AccelerationHandling/1(acceleration_world) -> KalmanFilter_dxdy/1
  Delay/1 -> UglyDataHandling/5(dxyOF_datin)
